simulink model "mysim"  (R2021a)
settings: Solver=ode23s  StartTime=0.0  StopTime=50  RelTol=1e-3
settings Model: Creator=camil  LastModifiedBy=camil

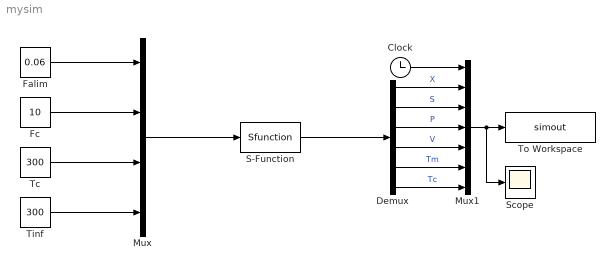
== system mysim ==
  Clock : Clock
  Demux : Demux  Outputs=6
  Falim : Constant  Value=0.06
  Fc : Constant  Value=10
  Mux : Mux
  Mux1 : Mux  Inputs=7
  S-Function : S-Function  FunctionName=Sfunction  SFunctionDeploymentMode=off  EnableBusSupport=off
  Scope : Scope
  Tc : Constant  Value=300
  Tinf : Constant  Value=300
  To Workspace : ToWorkspace  VariableName=simout  SampleTime=0.01
  wires:
  Falim/1 -> Mux/1
  Fc/1 -> Mux/2
  Mux/1 -> S-Function/1
  S-Function/1 -> Demux/1
  Demux/2 -> Mux1/3  "S"
  Demux/3 -> Mux1/4  "P"
  Clock/1 -> Mux1/1
  Mux1/1 -> Scope/1, To Workspace/1
  Demux/1 -> Mux1/2  "X"
  Demux/4 -> Mux1/5  "V"
  Demux/5 -> Mux1/6  "Tm"
  Demux/6 -> Mux1/7  "Tc"
  Tc/1 -> Mux/3
  Tinf/1 -> Mux/4
